simulink model "q_spg_pp"  (Simulink 10.3)
settings: Solver=ode4  StartTime=0.0  StopTime=inf  FixedStep=0.001  RelTol=1e-3  EnableMultiTasking=on
values from neighbouring files (symbols this model uses):
  ALPHA_LIM_ENABLE = 0    [setup_ip02_spg.m]
  ALPHA_MAX = 25    [setup_ip02_spg.m]
  ALPHA_MIN = - ALPHA_MAX    (= -25)    [setup_ip02_spg.m]
  K = [ 0 0 0 0 ]    [setup_ip02_spg.m]
  K_AMP = 1    [setup_ip02_spg.m]
  VMAX_DAC = 10    [setup_ip02_spg.m]
  wcf = 2 * pi * 10    (= 62.8318530718)    [setup_ip02_spg.m]
  X0 = [ 0; X0(2); 0; 0 ]    [setup_ip02_spg.m]
  X_LIM_ENABLE = 1    [setup_ip02_spg.m]
  X_MAX = 0.2    [setup_ip02_spg.m]
  X_MIN = - X_MAX    (= -0.2)    [setup_ip02_spg.m]
  zetaf = 0.9    [setup_ip02_spg.m]
undefined symbols (not defined in the file or in its folder): A, B, C, D, HIL, K_EC, K_EP, Lp, qc_get_step_size, VMAX_AMP
libraries: quarc_library x8, simulink_extras x3
settings Model: Creator=Mfotoohi  LastModifiedBy=MLevis  SimulationMode=external  ExtModeTrigDuration=10000
settings SolverCC: PositivePriorityOrder=on
settings DataIOCC: LimitDataPoints=on
settings OptimizationCC: InitFltsAndDblsToZero=on  LifeSpan=auto
settings DebuggingCC: SaveWithParameterizedLinksMsg=none  SolverPrmCheckMsg=warning  MultiTaskDSMMsg=warning  MultiTaskCondExecSysMsg=none
settings HardwareCC: ProdBitPerPointer=64  ProdBitPerSizeT=64  ProdBitPerPtrDiffT=64  ProdLargestAtomicFloat=Float  ProdIntDivRoundTo=Zero  ProdEndianess=LittleEndian  ProdWordSize=64  ProdHWDeviceType=Intel->x86-64 (Windows64)  TargetHWDeviceType=32-bit Generic
settings RTWCC: Description=QUARC Win64 Target Using Toolchain  SystemTargetFile=quarc_win64.tlc  TemplateMakefile=quarc_default_tmf  Toolchain=QUARC win64 | nmake (64-bit Windows)  BuildConfiguration=Faster Runs
settings STFCustomTargetCC: ConcurrentExecutionCompliant=on  UseToolchainInfoCompliant=on  SystemTargetFile=quarc_win64.tlc
settings GRTTargetCC: ParMdlRefBuildCompliant=off  CompOptLevelCompliant=off  MatFileLogging=off  CPPClassGenCompliant=off  ExtMode=on  ExtModeMexFile=quarc_comm

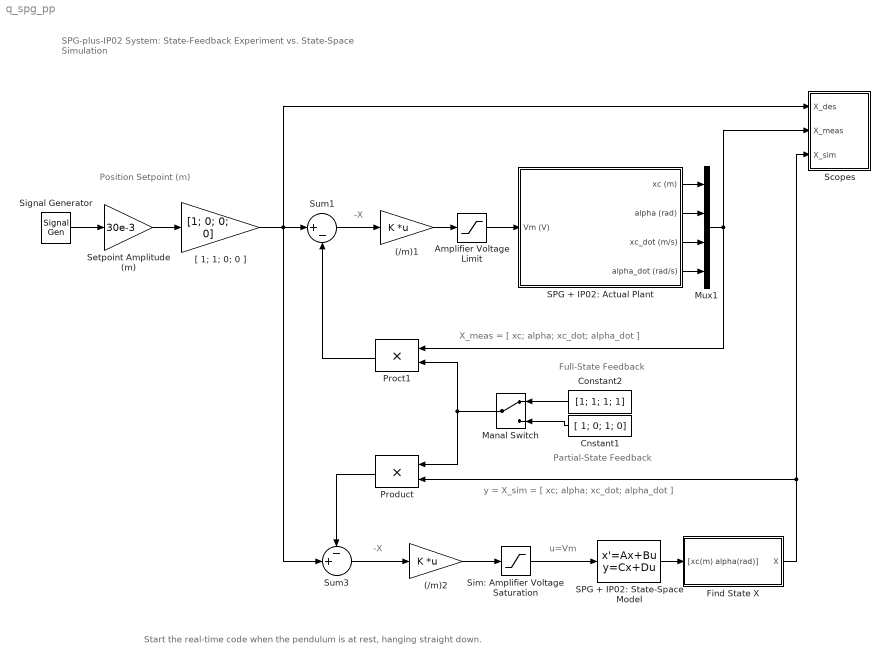
== system q_spg_pp ==
  note: u=Vm
  note: X_meas = [ xc; alpha; xc_dot; alpha_dot ]
  note: -X
  note: -X
  note: Position Setpoint (m)
  note: y = X_sim = [ xc; alpha; xc_dot; alpha_dot ]
  note: Full-State Feedback
  note: Partial-State Feedback
  note: SPG-plus-IP02 System: State-Feedback
      | Experiment vs. State-Space Simulation
  note: Start the real-time code when the pendulum is at rest, hanging straight down.
  (/m)1 : Gain  Gain=K  Multiplication=Matrix(K*u)  SaturateOnIntegerOverflow=on  OutDataTypeStr=Inherit: Same as input  ParamDataTypeStr=Inherit: Same as input
  (/m)2 : Gain  Gain=K  Multiplication=Matrix(K*u)  SaturateOnIntegerOverflow=on  OutDataTypeStr=Inherit: Same as input  ParamDataTypeStr=Inherit: Same as input
  Amplifier Voltage Limit : Saturate  UpperLimit=VMAX_AMP  LowerLimit=- VMAX_AMP
  Cnstant1 : Constant  Value=[ 1; 0; 1; 0]
  Constant2 : Constant  Value=[1; 1; 1; 1]
  Find State X : Subsystem
  Manal Switch : ManualSwitch
  Mux1 : Mux
  Proct1 : Product  InputSameDT=on  RndMeth=Zero  SaturateOnIntegerOverflow=on  OutDataTypeStr=Inherit: Same as first input
  Product : Product  InputSameDT=on  RndMeth=Zero  SaturateOnIntegerOverflow=on  OutDataTypeStr=Inherit: Same as first input
  SPG + IP02: Actual Plant : Subsystem
  SPG + IP02: State-Space Model : StateSpace  A=A  B=B  C=C  D=D  InitialCondition=X0
  Scopes : Subsystem
  Setpoint Amplitude (m) : Gain  Gain=30e-3  SaturateOnIntegerOverflow=on  OutDataTypeStr=Inherit: Same as input  ParamDataTypeStr=Inherit: Same as input
  Signal Generator : SignalGenerator  WaveForm=square  Frequency=0.1
  Sim: Amplifier Voltage Saturation : Saturate  UpperLimit=VMAX_AMP  LowerLimit=- VMAX_AMP
  Sum1 : Sum  Inputs=|+-  InputSameDT=on  SaturateOnIntegerOverflow=on  OutDataTypeStr=Inherit: Same as first input
  Sum3 : Sum  Inputs=-+|  InputSameDT=on  SaturateOnIntegerOverflow=on  OutDataTypeStr=Inherit: Same as first input
  "[ 1; 1; 0; 0 ]" : Gain  Gain=[1; 0; 0; 0]  SaturateOnIntegerOverflow=on  OutDataTypeStr=Inherit: Same as input  ParamDataTypeStr=Inherit: Same as input
  wires:
  SPG + IP02: Actual Plant/1(xc (m)) -> Mux1/1
  (/m)1/1 -> Amplifier Voltage Limit/1
  SPG + IP02: Actual Plant/2(alpha (rad)) -> Mux1/2
  SPG + IP02: Actual Plant/4(alpha_dot (rad/s)) -> Mux1/4
  Sim: Amplifier Voltage Saturation/1 -> SPG + IP02: State-Space Model/1
  (/m)2/1 -> Sim: Amplifier Voltage Saturation/1
  Sum3/1 -> (/m)2/1
  Sum1/1 -> (/m)1/1
  "[ 1; 1; 0; 0 ]"/1 -> Sum1/1, Scopes/1(X_des), Sum3/2
  Mux1/1 -> Scopes/2(X_meas), Proct1/1
  Setpoint Amplitude (m)/1 -> "[ 1; 1; 0; 0 ]"/1
  SPG + IP02: Actual Plant/3(xc_dot (m/s)) -> Mux1/3
  Signal Generator/1 -> Setpoint Amplitude (m)/1
  Constant2/1 -> Manal Switch/1
  Cnstant1/1 -> Manal Switch/2
  Manal Switch/1 -> Proct1/2, Product/1
  Proct1/1 -> Sum1/2
  Product/1 -> Sum3/1
  Amplifier Voltage Limit/1 -> SPG + IP02: Actual Plant/1(Vm (V))
  SPG + IP02: State-Space Model/1 -> Find State X/1("[xc(m) alpha(rad)]")
  Find State X/1(X) -> Scopes/3(X_sim), Product/2

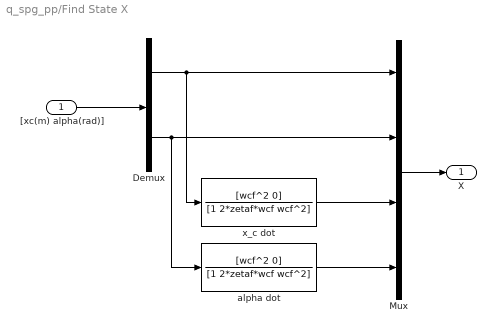
== system q_spg_pp/Find State X ==
  "[xc(m) alpha(rad)]" : Inport
  Demux : Demux  Outputs=2
  Mux : Mux
  alpha dot : TransferFcn  Numerator=[wcf^2 0]  Denominator=[1 2*zetaf*wcf wcf^2]
  x_c dot : TransferFcn  Numerator=[wcf^2 0]  Denominator=[1 2*zetaf*wcf wcf^2]
  X : Outport
  wires:
  Mux/1 -> X/1
  x_c dot/1 -> Mux/3
  alpha dot/1 -> Mux/4
  "[xc(m) alpha(rad)]"/1 -> Demux/1
  Demux/1 -> Mux/1, x_c dot/1
  Demux/2 -> Mux/2, alpha dot/1

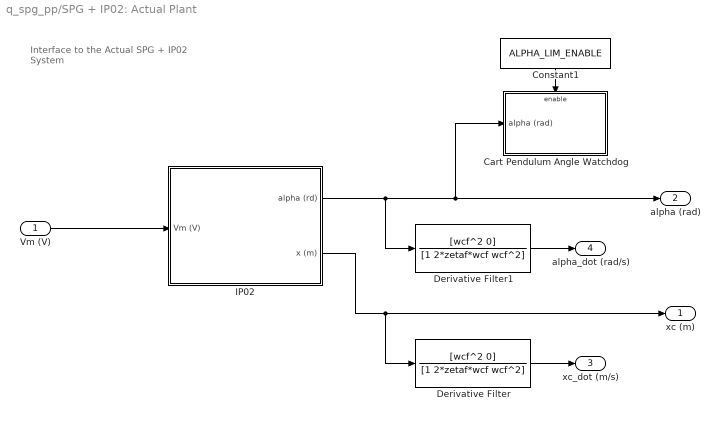
== system q_spg_pp/SPG + IP02: Actual Plant ==
  note: Interface to the Actual
      | SPG + IP02 System
  Vm (V) : Inport
  Cart Pendulum Angle Watchdog : Subsystem  TreatAsAtomicUnit=on
  Constant1 : Constant  Value=ALPHA_LIM_ENABLE
  Derivative Filter : TransferFcn  Numerator=[wcf^2 0]  Denominator=[1 2*zetaf*wcf wcf^2]
  Derivative Filter1 : TransferFcn  Numerator=[wcf^2 0]  Denominator=[1 2*zetaf*wcf wcf^2]
  IP02 : Subsystem
  xc (m) : Outport  InitialOutput=0
  alpha (rad) : Outport  Port=2  InitialOutput=0
  xc_dot (m/s) : Outport  Port=3  InitialOutput=0
  alpha_dot (rad/s) : Outport  Port=4  InitialOutput=0
  wires:
  Vm (V)/1 -> IP02/1(Vm (V))
  IP02/2(x (m)) -> xc (m)/1, Derivative Filter/1
  Derivative Filter1/1 -> alpha_dot (rad/s)/1
  IP02/1(alpha (rd)) -> Derivative Filter1/1, alpha (rad)/1, Cart Pendulum Angle Watchdog/1(alpha (rad))
  Derivative Filter/1 -> xc_dot (m/s)/1
  Constant1/1 -> Cart Pendulum Angle Watchdog/Enable

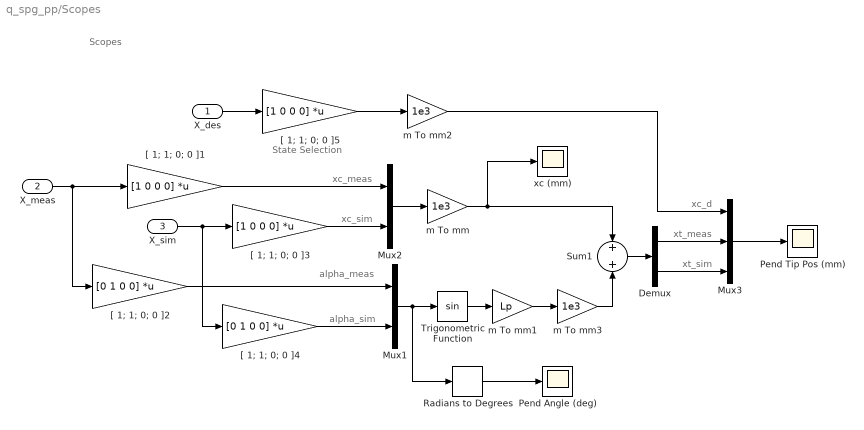
== system q_spg_pp/Scopes ==
  note: xc_meas
  note: State Selection
  note: alpha_meas
  note: alpha_sim
  note: xc_sim
  note: xc_d
  note: Scopes
  note: xt_sim
  note: xt_meas
  X_des : Inport
  X_meas : Inport  Port=2
  X_sim : Inport  Port=3
  Demux : Demux  Outputs=2
      settings: DisplayOption=none
  Mux1 : Mux  Inputs=2
  Mux2 : Mux  Inputs=2
  Mux3 : Mux  Inputs=3
  Pend Angle (deg) : Scope
  Pend Tip Pos (mm) : Scope
  Radians to Degrees : simulink_extras/Transformations/Radians to Degrees
  Sum1 : Sum  Inputs=+|+  InputSameDT=on  SaturateOnIntegerOverflow=on  OutDataTypeStr=Inherit: Same as first input
  Trigonometric Function : Trigonometry
  "[ 1; 1; 0; 0 ]1" : Gain  Gain=[1 0 0 0]  Multiplication=Matrix(K*u)  SaturateOnIntegerOverflow=on  OutDataTypeStr=Inherit: Same as input  ParamDataTypeStr=Inherit: Same as input
  "[ 1; 1; 0; 0 ]2" : Gain  Gain=[0 1 0 0]  Multiplication=Matrix(K*u)  SaturateOnIntegerOverflow=on  OutDataTypeStr=Inherit: Same as input  ParamDataTypeStr=Inherit: Same as input
  "[ 1; 1; 0; 0 ]3" : Gain  Gain=[1 0 0 0]  Multiplication=Matrix(K*u)  SaturateOnIntegerOverflow=on  OutDataTypeStr=Inherit: Same as input  ParamDataTypeStr=Inherit: Same as input
  "[ 1; 1; 0; 0 ]4" : Gain  Gain=[0 1 0 0]  Multiplication=Matrix(K*u)  SaturateOnIntegerOverflow=on  OutDataTypeStr=Inherit: Same as input  ParamDataTypeStr=Inherit: Same as input
  "[ 1; 1; 0; 0 ]5" : Gain  Gain=[1 0 0 0]  Multiplication=Matrix(K*u)  SaturateOnIntegerOverflow=on  OutDataTypeStr=Inherit: Same as input  ParamDataTypeStr=Inherit: Same as input
  m To mm : Gain  Gain=1e3  SaturateOnIntegerOverflow=on  OutDataTypeStr=Inherit: Same as input  ParamDataTypeStr=Inherit: Same as input
  m To mm1 : Gain  Gain=Lp  SaturateOnIntegerOverflow=on  OutDataTypeStr=Inherit: Same as input  ParamDataTypeStr=Inherit: Same as input
  m To mm2 : Gain  Gain=1e3  SaturateOnIntegerOverflow=on  OutDataTypeStr=Inherit: Same as input  ParamDataTypeStr=Inherit: Same as input
  m To mm3 : Gain  Gain=1e3  SaturateOnIntegerOverflow=on  OutDataTypeStr=Inherit: Same as input  ParamDataTypeStr=Inherit: Same as input
  xc (mm) : Scope
  wires:
  Mux2/1 -> m To mm/1
  m To mm/1 -> Sum1/1, xc (mm)/1
  X_des/1 -> "[ 1; 1; 0; 0 ]5"/1
  X_meas/1 -> "[ 1; 1; 0; 0 ]1"/1, "[ 1; 1; 0; 0 ]2"/1
  Mux1/1 -> Trigonometric Function/1, Radians to Degrees/1
  X_sim/1 -> "[ 1; 1; 0; 0 ]3"/1, "[ 1; 1; 0; 0 ]4"/1
  "[ 1; 1; 0; 0 ]3"/1 -> Mux2/2
  m To mm1/1 -> m To mm3/1
  Trigonometric Function/1 -> m To mm1/1
  m To mm3/1 -> Sum1/2
  "[ 1; 1; 0; 0 ]1"/1 -> Mux2/1
  "[ 1; 1; 0; 0 ]5"/1 -> m To mm2/1
  m To mm2/1 -> Mux3/1
  Mux3/1 -> Pend Tip Pos (mm)/1
  Sum1/1 -> Demux/1
  "[ 1; 1; 0; 0 ]4"/1 -> Mux1/2
  "[ 1; 1; 0; 0 ]2"/1 -> Mux1/1
  Demux/1 -> Mux3/2
  Demux/2 -> Mux3/3
  Radians to Degrees/1 -> Pend Angle (deg)/1

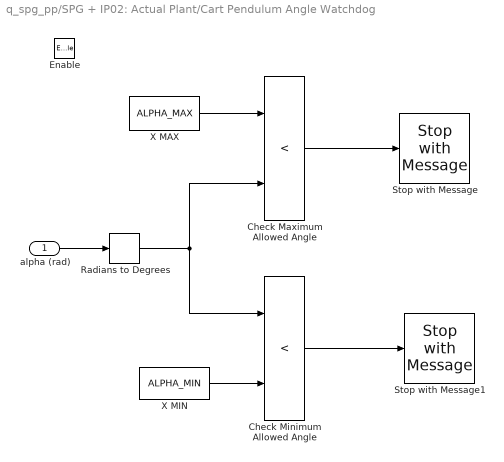
== system q_spg_pp/SPG + IP02: Actual Plant/Cart Pendulum Angle Watchdog ==
  alpha (rad) : Inport
  Enable : EnablePort
  Check Maximum Allowed Angle : RelationalOperator  Operator=<  RndMeth=Nearest  InputSameDT=on
  Check Minimum Allowed Angle : RelationalOperator  Operator=<  RndMeth=Nearest  InputSameDT=on
  Radians to Degrees : simulink_extras/Transformations/Radians to Degrees
  Stop with Message : quarc_library/Sinks/Error Handling/Stop with Message  message_type=Fixed error message  message_icon=Error  message=Maximum Angle Reached.
  Stop with Message1 : quarc_library/Sinks/Error Handling/Stop with Message  message_type=Fixed error message  message_icon=Error  message=Maximum Angle Reached.
  X MAX : Constant  Value=ALPHA_MAX
  X MIN : Constant  Value=ALPHA_MIN
  wires:
  X MAX/1 -> Check Maximum Allowed Angle/1
  Check Minimum Allowed Angle/1 -> Stop with Message1/1
  X MIN/1 -> Check Minimum Allowed Angle/2
  alpha (rad)/1 -> Radians to Degrees/1
  Check Maximum Allowed Angle/1 -> Stop with Message/1
  Radians to Degrees/1 -> Check Maximum Allowed Angle/2, Check Minimum Allowed Angle/1

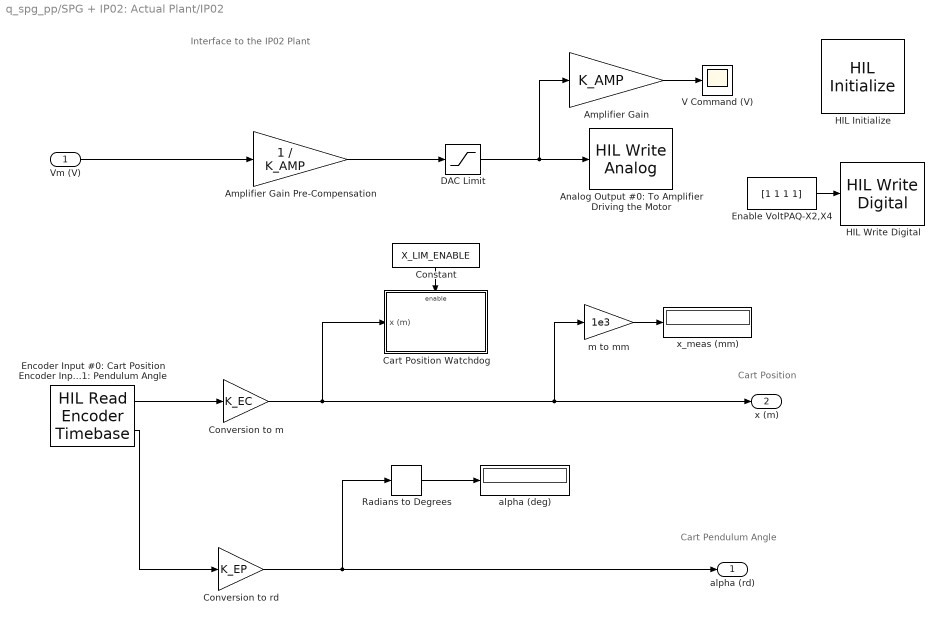
== system q_spg_pp/SPG + IP02: Actual Plant/IP02 ==
  note: Cart Pendulum Angle
  note: Cart Position
  note: Interface to the IP02 Plant
  Vm (V) : Inport
  Amplifier Gain : Gain  Gain=K_AMP  SaturateOnIntegerOverflow=on  OutDataTypeStr=Inherit: Same as input  ParamDataTypeStr=Inherit: Same as input
  Amplifier Gain Pre-Compensation : Gain  Gain=1 / K_AMP  SaturateOnIntegerOverflow=on  OutDataTypeStr=Inherit: Same as input  ParamDataTypeStr=Inherit: Same as input
  Analog Output #0: To Amplifier Driving the Motor : quarc_library/Data Acquisition/Generic/Immediate I//O/HIL Write Analog  Tag=unassigned  object_name=HIL-1  channels=0  sample_time=-1  active=on  vector_input=on
  Cart Position Watchdog : Subsystem  TreatAsAtomicUnit=on
  Constant : Constant  Value=X_LIM_ENABLE
  Conversion to m : Gain  Gain=K_EC  SaturateOnIntegerOverflow=on  OutDataTypeStr=Inherit: Same as input  ParamDataTypeStr=Inherit: Same as input
  Conversion to rd : Gain  Gain=K_EP  SaturateOnIntegerOverflow=on  OutDataTypeStr=Inherit: Same as input  ParamDataTypeStr=Inherit: Same as input
  DAC Limit : Saturate  UpperLimit=VMAX_DAC  LowerLimit=- VMAX_DAC
  Enable VoltPAQ-X2,X4 : Constant  Value=[1 1 1 1]
  Encoder Input #0: Cart Position Encoder Input #1: Pendulum Angle : quarc_library/Data Acquisition/Generic/Timebases/HIL Read Encoder Timebase  Tag=unassigned  object_name=HIL-1  clock=0  channels=[0 1]  samples_in_buffer=max(ceil(1/qc_get_step_size), 1)  active=on  vector_output=off  data_type_mode=Inherit via back propagation  data_type=double
  HIL Initialize : quarc_library/Data Acquisition/Generic/Configuration/HIL Initialize  object_name=HIL-1  board_type=q2_usb  board_number=0  board_options=d0=digital;d1=digital;led=auto;update_rate=normal  exclusive=off  active=off  hardware_clocks=[0:2]  clock_modes=[]  initial_clock_frequencies=[]  set_clock_params_at_start=off  set_clock_params_at_switch_in=off  set_clock_frequencies_at_start=off  set_clock_frequencies_at_switch_in=off  analog_input_channels=[0:1]  analog_input_maximums=10  analog_input_minimums=-10  set_analog_input_params_at_start=on  set_analog_input_params_at_switch_in=off  analog_output_channels=[0:1]  analog_output_maximums=10  analog_output_minimums=-10  initial_analog_outputs=[0]  final_analog_outputs=[0]  watchdog_analog_outputs=0  set_analog_output_params_at_start=on  set_analog_output_params_at_switch_in=off  set_analog_outputs_at_start=on  set_analog_outputs_at_switch_in=off  set_analog_outputs_at_terminate=on  set_analog_outputs_at_switch_out=off  set_analog_outputs_on_watchdog=off  digital_input_channels=[]  digital_output_channels=[0:7]  digital_output_configuration=[]  initial_digital_outputs=[0]  final_digital_outputs=[0]  watchdog_digital_outputs=[0]  set_digital_output_params_at_start=off  set_digital_output_params_at_switch_in=off  set_digital_outputs_at_start=on  set_digital_outputs_at_switch_in=off  set_digital_outputs_at_terminate=on  set_digital_outputs_at_switch_out=off  set_digital_outputs_on_watchdog=off  encoder_channels=[0:1]  quadrature=[4]  encoder_filter_frequency=[]  initial_encoder_counts=[0]  set_encoder_params_at_start=on  set_encoder_params_at_switch_in=off  set_encoder_counts_at_start=on  set_encoder_counts_at_switch_in=off  pwm_channels=[]  pwm_modes=[0]  pwm_frequency=1/0.020  pwm_configuration=[]  pwm_alignment=[]  pwm_polarity=[]  pwm_leading_deadband=[]  pwm_trailing_deadband=[]  initial_pwm_outputs=[0]  final_pwm_outputs=[0]  watchdog_pwm_outputs=[0]  set_pwm_params_at_start=on  set_pwm_params_at_switch_in=off  set_pwm_outputs_at_start=on  set_pwm_outputs_at_switch_in=off  set_pwm_outputs_at_terminate=on  set_pwm_outputs_at_switch_out=off  set_pwm_outputs_on_watchdog=off  other_output_channels=[]  initial_other_outputs=[]  final_other_outputs=[]  watchdog_other_outputs=[]  set_other_outputs_at_start=off  set_other_outputs_at_switch_in=off  set_other_outputs_at_terminate=off  set_other_outputs_at_switch_out=off  set_other_outputs_on_watchdog=off
  HIL Write Digital : quarc_library/Data Acquisition/Generic/Immediate I//O/HIL Write Digital  object_name=HIL-1  channels=[0:3]  sample_time=-1  active=off  vector_input=on
      settings: SourceProductName=QUARC Targets
  Radians to Degrees : simulink_extras/Transformations/Radians to Degrees
  V Command (V) : Scope
  alpha (deg) : Display
      settings: Decimation=100
  m to mm : Gain  Gain=1e3  SaturateOnIntegerOverflow=on  OutDataTypeStr=Inherit: Same as input  ParamDataTypeStr=Inherit: Same as input
  x_meas (mm) : Display
      settings: Decimation=100
  alpha (rd) : Outport  InitialOutput=0
  x (m) : Outport  Port=2  InitialOutput=0
  wires:
  Encoder Input #0: Cart Position Encoder Input #1: Pendulum Angle/1 -> Conversion to m/1
  Conversion to m/1 -> Cart Position Watchdog/1(x (m)), x (m)/1, m to mm/1
  Amplifier Gain Pre-Compensation/1 -> DAC Limit/1
  m to mm/1 -> x_meas (mm)/1
  Encoder Input #0: Cart Position Encoder Input #1: Pendulum Angle/2 -> Conversion to rd/1
  Radians to Degrees/1 -> alpha (deg)/1
  Conversion to rd/1 -> Radians to Degrees/1, alpha (rd)/1
  Constant/1 -> Cart Position Watchdog/Enable
  DAC Limit/1 -> Analog Output #0: To Amplifier Driving the Motor/1, Amplifier Gain/1
  Vm (V)/1 -> Amplifier Gain Pre-Compensation/1
  Amplifier Gain/1 -> V Command (V)/1
  Enable VoltPAQ-X2,X4/1 -> HIL Write Digital/1

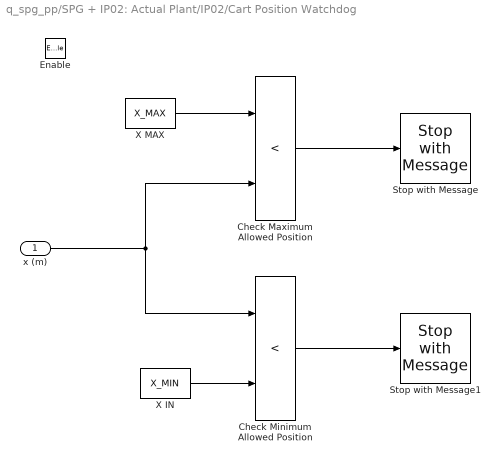
== system q_spg_pp/SPG + IP02: Actual Plant/IP02/Cart Position Watchdog ==
  x (m) : Inport
  Enable : EnablePort
  Check Maximum Allowed Position : RelationalOperator  Operator=<  RndMeth=Nearest  InputSameDT=on
  Check Minimum Allowed Position : RelationalOperator  Operator=<  RndMeth=Nearest  InputSameDT=on
  Stop with Message : quarc_library/Sinks/Error Handling/Stop with Message  message_type=Fixed error message  message_icon=Error  message=Maximum Limit Reached.
  Stop with Message1 : quarc_library/Sinks/Error Handling/Stop with Message  message_type=Fixed error message  message_icon=Error  message=Minimum Limit Reached.
  X IN : Constant  Value=X_MIN
  X MAX : Constant  Value=X_MAX
  wires:
  Check Maximum Allowed Position/1 -> Stop with Message/1
  x (m)/1 -> Check Minimum Allowed Position/1, Check Maximum Allowed Position/2
  X IN/1 -> Check Minimum Allowed Position/2
  Check Minimum Allowed Position/1 -> Stop with Message1/1
  X MAX/1 -> Check Maximum Allowed Position/1
